simulink model "Sin_model_cs"  (R2021b)
settings: Solver=ode15s  StartTime=0.0  StopTime=4  MaxStep=1e-5  RelTol=2.22045e-14  AbsTol=1e-20
values from neighbouring files (symbols this model uses):
  K_vco = 250    [parameters.m]
  omega_vco_free = 0    [parameters.m]
  tau_1 = 0.0186    [parameters.m]
  tau_2 = 0.0225    [parameters.m]
libraries: simulink x1
settings Model: Creator=Vogal  LastModifiedBy=milich
settings SolverCC: InitialStep=1e-20  AlgebraicLoopSolver=TrustRegion
settings DataIOCC: ReturnWorkspaceOutputs=off
settings DebuggingCC: SFMachineParentedDataDiag=warning  ArithmeticOperatorsInVariantConditions=warning
settings SFSimCC: SimUseLocalCustomCode=off  CustomCodeUndefinedFunction=UseInterfaceOnly
settings RTWCC: RTWUseLocalCustomCode=off

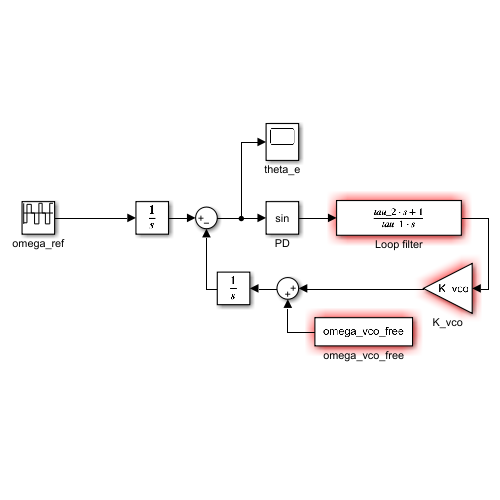
[thumbnail: Simulink's stored preview of the top-level diagram]
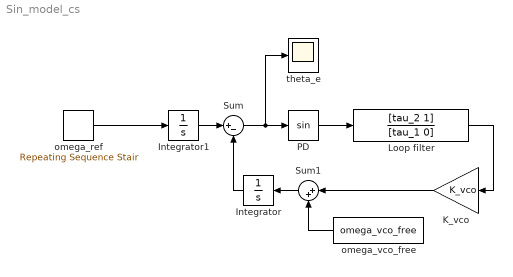
== system Sin_model_cs ==
  Integrator : Integrator
  Integrator1 : Integrator
  K_vco : Gain  Gain=K_vco
  Loop filter : TransferFcn  Numerator=[tau_2 1]  Denominator=[tau_1 0]
  PD : Trigonometry
  Sum : Sum  Inputs=|+-
  Sum1 : Sum  Inputs=|++
  omega_ref : simulink/Sources/Repeating Sequence Stair  OutValues=[-213.39 213.39 0 -239.7 239.7 0 -240.43 240.43].'  tsamp=0.5  OutMin=[]  OutMax=[]  OutDataTypeStr=double  OutputDataTypeScalingMode=double  OutDataType=fixdt(0,8)  ConRadixGroup=Best Precision: Vector-wise  OutScaling=2^-12
  "omega_vco_free " : Constant  Value=omega_vco_free
  theta_e : Scope
  wires:
  PD/1 -> Loop filter/1
  Loop filter/1 -> K_vco/1
  K_vco/1 -> Sum1/1
  "omega_vco_free "/1 -> Sum1/2
  Sum1/1 -> Integrator/1
  Integrator/1 -> Sum/2
  Integrator1/1 -> Sum/1
  Sum/1 -> theta_e/1, PD/1
  omega_ref/1 -> Integrator1/1
